simulink model "SPGF_FSK_0000_R2019b"  (R2019b)
settings: Solver=ode3  SolverName=ode4  StartTime=0.0  StopTime=1.4  FixedStep=50e-6/50  RelTol=1e-3  EnableMultiTasking=on
undefined symbols (not defined in the file): D11, Delta
libraries: powerlib x2544, powerlib_meascontrol x204, simulink x24
(part 14 of 33)

== system SPGF_FSK_0000_R2019b/W13/DPL ==
  Ccs2/1 : powerlib/Elements/Series RLC Branch  LConnTagsString=__new0  RConnTagsString=__new0  BranchType=R  Resistance=-Rg_matrix(3,4)*2  Inductance=1e-3  SetiL0=off  InitialCurrent=0  Capacitance=Rg_matrix(3,4)*2  Setx0=off  InitialVoltage=0  Measurements=None
  Ccs2/3 : powerlib/Elements/Series RLC Branch  LConnTagsString=__new0  RConnTagsString=__new0  BranchType=R  Resistance=-Rg_matrix(3,4)*2  Inductance=1e-3  SetiL0=off  InitialCurrent=0  Capacitance=Rg_matrix(3,4)*2  Setx0=off  InitialVoltage=0  Measurements=None
  Ccs3/1 : powerlib/Elements/Series RLC Branch  LConnTagsString=__new0  RConnTagsString=__new0  BranchType=R  Resistance=-Rg_matrix(5,6)*2  Inductance=1e-3  SetiL0=off  InitialCurrent=0  Capacitance=-C_matrix(5,6)/2  Setx0=off  InitialVoltage=0  Measurements=None
  Ccs3/3 : powerlib/Elements/Series RLC Branch  LConnTagsString=__new0  RConnTagsString=__new0  BranchType=R  Resistance=-Rg_matrix(5,6)*2  Inductance=1e-3  SetiL0=off  InitialCurrent=0  Capacitance=-C_matrix(5,6)/2  Setx0=off  InitialVoltage=0  Measurements=None
  DPL : powerlib/Elements/Distributed Parameters Line  Phases=6  Length=LineLength  Frequency=Frequency  Resistance=R_matrix  Inductance=L_matrix  Capacitance=C_matrix  x1=[-8.15e-05 -1.48873142828454 0 -11.7861642745277 0 4676.68792805612 0;-8.1e-05 -1.48913663578964 0 -11.7892921080622 0 4676.29069613494 0;-8.05e-05 -1.48954180655177 0 -11.7924196507075 0 4675.89334883091 0;-8e-05 -1.48994694056093 0 -11.7955469023866 0 4675.49588615384 0;-7.95e-05 -1.49035203780712 0 -11.7986738630222 0 4675.09830811353 0;-7.9e-05 -1.49075709828036 0 -11.8018005325372 0 4674.70061471979 0;-7.85e-05 -1.49116212197063 0 -11.8049269108544 0 4674.30280598244 0;-7.8e-05 -1.49156710886795 0 -11.8080529978968 0 4673.90488191129 0;-7.75e-05 -1.49197205896233 0 -11.8111787935871 0 4673.50684251616 0;-7.7e-05 -1.49237697224378 0 -11.8143042978483 0 4673.10868780687 0;-7.65e-05 -1.49278184870229 0 -11.8174295106032 0 4672.71041779325 0;-7.6e-05 -1.4931866883279 0 -11.8205544317747 0 4672.31203248511 0;-7.55e-05 -1.4935914911106 0 -11.8236790612857 0 4671.9135318923 0;-7.5e-05 -1.4939962570404 0 -11.8268033990591 0 4671.51491602465 0;-7.45e-05 -1.49440098610733 0 -11.8299274450179 0 4671.11618489198 0;-7.4e-05 -1.49480567830139 0 -11.8330511990848 0 4670.71733850414 0;-7.35e-05 -1.49521033361259 0 -11.836174661183 0 4670.31837687097 0;-7.3e-05 -1.49561495203097 0 -11.8392978312353 0 4669.91930000232 0;-7.25e-05 -1.49601953354652 0 -11.8424207091646 0 4669.52010790802 0;-7.2e-05 -1.49642407814927 0 -11.8455432948938 0 4669.12080059794 0;-7.15e-05 -1.49682858582923 0 -11.848665588346 0 4668.72137808191 0;-7.1e-05 -1.49723305657643 0 -11.8517875894441 0 4668.3218403698 0;-7.05e-05 -1.49763749038089 0 -11.8549092981111 0 4667.92218747147 0;-7e-05 -1.49804188723262 0 -11.8580307142699 0 4667.52241939678 0;-6.95e-05 -1.49844624712165 0 -11.8611518378435 0 4667.12253615559 0;-6.9e-05 -1.498850570038 0 -11.864272668755 0 4666.72253775776 0;-6.85e-05 -1.4992548559717 0 -11.8673932069272 0 4666.32242421317 0;-6.8e-05 -1.49965910491276 0 -11.8705134522833 0 4665.9221955317 0;-6.75e-05 -1.50006331685122 0 -11.8736334047461 0 4665.5218517232 0;-6.7e-05 -1.5004674917771 0 -11.8767530642388 0 4665.12139279757 0;-6.65e-05 -1.50087162968043 0 -11.8798724306844 0 4664.72081876468 0;-6.6e-05 -1.50127573055124 0 -11.8829915040059 0 4664.32012963442 0;-6.55e-05 -1.50167979437955 0 -11.8861102841263 0 4663.91932541667 0;-6.5e-05 -1.5020838211554 0 -11.8892287709687 0 4663.51840612133 0;-6.45e-05 -1.50248781086881 0 -11.8923469644561 0 4663.11737175828 0;-6.4e-05 -1.50289176350983 0 -11.8954648645117 0 4662.71622233743 0;-6.35e-05 -1.50329567906848 0 -11.8985824710584 0 4662.31495786866 0;-6.3e-05 -1.50369955753479 0 -11.9016997840193 0 4661.91357836188 0;-6.25e-05 -1.5041033988988 0 -11.9048168033176 0 4661.512083827 0;-6.2e-05 -1.50450720315056 0 -11.9079335288763 0 4661.11047427391 0;-6.15e-05 -1.50491097028008 0 -11.9110499606185 0 4660.70874971254 0;-6.1e-05 -1.50531470027741 0 -11.9141660984673 0 4660.30691015278 0;-6.05e-05 -1.50571839313259 0 -11.9172819423459 0 4659.90495560456 0;-6e-05 -1.50612204883566 0 -11.9203974921773 0 4659.5028860778 0;-5.95e-05 -1.50652566737666 0 -11.9235127478848 0 4659.10070158241 0;-5.9e-05 -1.50692924874563 0 -11.9266277093913 0 4658.69840212832 0;-5.85e-05 -1.50733279293261 0 -11.9297423766201 0 4658.29598772545 0;-5.8e-05 -1.50773629992764 0 -11.9328567494943 0 4657.89345838374 0;-5.75e-05 -1.50813976972077 0 -11.935970827937 0 4657.49081411311 0;-5.7e-05 -1.50854320230205 0 -11.9390846118715 0 4657.08805492351 0;-5.65e-05 -1.50894659766151 0 -11.9421981012209 0 4656.68518082486 0;-5.6e-05 -1.5093499557892 0 -11.9453112959083 0 4656.28219182711 0;-5.55e-05 -1.50975327667518 0 -11.948424195857 0 4655.8790879402 0;-5.5e-05 -1.51015656030949 0 -11.9515368009902 0 4655.47586917409 0;-5.45e-05 -1.51055980668219 0 -11.954649111231 0 4655.0725355387 0;-5.4e-05 -1.51096301578331 0 -11.9577611265026 0 4654.66908704401 0;-5.35e-05 -1.51136618760291 0 -11.9608728467284 0 4654.26552369996 0;-5.3e-05 -1.51176932213105 0 -11.9639842718314 0 4653.86184551652 0;-5.25e-05 -1.51217241935778 0 -11.9670954017349 0 ...(+8261 chars)]  x2=[-8.15e-05 -1.48162132976478 0 -11.6914851169798 0 4744.49609233801 0;-8.1e-05 -1.48204386266957 0 -11.694778370435 0 4744.09779479294 0;-8.05e-05 -1.48246635900639 0 -11.6980713353332 0 4743.69938019196 0;-8e-05 -1.48288881876481 0 -11.701364011593 0 4743.30084854488 0;-7.95e-05 -1.48331124193443 0 -11.7046563991333 0 4742.90219986155 0;-7.9e-05 -1.4837336285048 0 -11.7079484978727 0 4742.5034341518 0;-7.85e-05 -1.48415597846552 0 -11.7112403077301 0 4742.10455142546 0;-7.8e-05 -1.48457829180615 0 -11.7145318286242 0 4741.70555169239 0;-7.75e-05 -1.48500056851628 0 -11.7178230604738 0 4741.30643496242 0;-7.7e-05 -1.48542280858549 0 -11.7211140031977 0 4740.9072012454 0;-7.65e-05 -1.48584501200337 0 -11.7244046567148 0 4740.50785055119 0;-7.6e-05 -1.48626717875949 0 -11.7276950209437 0 4740.10838288964 0;-7.55e-05 -1.48668930884343 0 -11.7309850958034 0 4739.70879827059 0;-7.5e-05 -1.48711140224479 0 -11.7342748812126 0 4739.30909670393 0;-7.45e-05 -1.48753345895314 0 -11.7375643770902 0 4738.90927819949 0;-7.4e-05 -1.48795547895808 0 -11.7408535833549 0 4738.50934276716 0;-7.35e-05 -1.48837746224919 0 -11.7441424999258 0 4738.1092904168 0;-7.3e-05 -1.48879940881605 0 -11.7474311267215 0 4737.70912115827 0;-7.25e-05 -1.48922131864826 0 -11.750719463661 0 4737.30883500146 0;-7.2e-05 -1.48964319173541 0 -11.7540075106631 0 4736.90843195624 0;-7.15e-05 -1.49006502806709 0 -11.7572952676467 0 4736.50791203249 0;-7.1e-05 -1.49048682763288 0 -11.7605827345307 0 4736.10727524009 0;-7.05e-05 -1.49090859042239 0 -11.763869911234 0 4735.70652158893 0;-7e-05 -1.49133031642521 0 -11.7671567976753 0 4735.30565108889 0;-6.95e-05 -1.49175200563092 0 -11.7704433937737 0 4734.90466374987 0;-6.9e-05 -1.49217365802912 0 -11.7737296994481 0 4734.50355958176 0;-6.85e-05 -1.49259527360942 0 -11.7770157146173 0 4734.10233859446 0;-6.8e-05 -1.49301685236141 0 -11.7803014392004 0 4733.70100079787 0;-6.75e-05 -1.49343839427468 0 -11.7835868731161 0 4733.29954620188 0;-6.7e-05 -1.49385989933883 0 -11.7868720162835 0 4732.89797481641 0;-6.65e-05 -1.49428136754348 0 -11.7901568686214 0 4732.49628665136 0;-6.6e-05 -1.4947027988782 0 -11.7934414300489 0 4732.09448171665 0;-6.55e-05 -1.49512419333261 0 -11.7967257004849 0 4731.69256002219 0;-6.5e-05 -1.49554555089632 0 -11.8000096798484 0 4731.29052157789 0;-6.45e-05 -1.49596687155891 0 -11.8032933680583 0 4730.88836639368 0;-6.4e-05 -1.49638815531 0 -11.8065767650336 0 4730.48609447948 0;-6.35e-05 -1.49680940213919 0 -11.8098598706933 0 4730.08370584521 0;-6.3e-05 -1.4972306120361 0 -11.8131426849564 0 4729.6812005008 0;-6.25e-05 -1.49765178499031 0 -11.8164252077419 0 4729.27857845619 0;-6.2e-05 -1.49807292099146 0 -11.8197074389688 0 4728.87583972131 0;-6.15e-05 -1.49849402002913 0 -11.8229893785561 0 4728.47298430609 0;-6.1e-05 -1.49891508209295 0 -11.8262710264228 0 4728.07001222048 0;-6.05e-05 -1.49933610717251 0 -11.829552382488 0 4727.66692347442 0;-6e-05 -1.49975709525745 0 -11.8328334466706 0 4727.26371807785 0;-5.95e-05 -1.50017804633736 0 -11.8361142188898 0 4726.86039604073 0;-5.9e-05 -1.50059896040186 0 -11.8393946990646 0 4726.456957373 0;-5.85e-05 -1.50101983744056 0 -11.8426748871141 0 4726.05340208462 0;-5.8e-05 -1.50144067744309 0 -11.8459547829572 0 4725.64973018554 0;-5.75e-05 -1.50186148039905 0 -11.8492343865132 0 4725.24594168573 0;-5.7e-05 -1.50228224629806 0 -11.852513697701 0 4724.84203659516 0;-5.65e-05 -1.50270297512975 0 -11.8557927164397 0 4724.43801492378 0;-5.6e-05 -1.50312366688373 0 -11.8590714426485 0 4724.03387668156 0;-5.55e-05 -1.50354432154961 0 -11.8623498762464 0 4723.62962187848 0;-5.5e-05 -1.50396493911703 0 -11.8656280171526 0 4723.22525052451 0;-5.45e-05 -1.5043855195756 0 -11.8689058652861 0 4722.82076262963 0;-5.4e-05 -1.50480606291495 0 -11.8721834205661 0 4722.41615820382 0;-5.35e-05 -1.50522656912469 0 -11.8754606829118 0 4722.01143725705 0;-5.3e-05 -1.50564703819446 0 -11.8787376522422 0 4721.60659979933 0;-5.25e-05 -1.50606747011388 0 -11.8820143284765 0 ...(+8265 chars)]  x3=[-8.15e-05 0.0158008018941895 0 -0.497557667568893 0 442.095796396926 0;-8.1e-05 0.0157969192286376 0 -0.497893185344398 0 442.062522662758 0;-8.05e-05 0.0157930361733123 0 -0.498228690834881 0 442.029238021135 0;-8e-05 0.0157891527283095 0 -0.498564184032065 0 441.995942472877 0;-7.95e-05 0.015785268893725 0 -0.49889966492767 0 441.962636018807 0;-7.9e-05 0.0157813846696546 0 -0.499235133513419 0 441.929318659746 0;-7.85e-05 0.0157775000561941 0 -0.499570589781035 0 441.895990396516 0;-7.8e-05 0.0157736150534395 0 -0.499906033722241 0 441.86265122994 0;-7.75e-05 0.0157697296614864 0 -0.50024146532876 0 441.82930116084 0;-7.7e-05 0.0157658438804309 0 -0.500576884592316 0 441.795940190038 0;-7.65e-05 0.0157619577103688 0 -0.500912291504632 0 441.762568318359 0;-7.6e-05 0.015758071151396 0 -0.501247686057433 0 441.729185546626 0;-7.55e-05 0.0157541842036083 0 -0.501583068242443 0 441.695791875661 0;-7.5e-05 0.0157502968671017 0 -0.501918438051386 0 441.66238730629 0;-7.45e-05 0.0157464091419722 0 -0.502253795475989 0 441.628971839336 0;-7.4e-05 0.0157425210283155 0 -0.502589140507976 0 441.595545475624 0;-7.35e-05 0.0157386325262278 0 -0.502924473139073 0 441.562108215979 0;-7.3e-05 0.0157347436358048 0 -0.503259793361006 0 441.528660061225 0;-7.25e-05 0.0157308543571426 0 -0.503595101165502 0 441.495201012189 0;-7.2e-05 0.0157269646903371 0 -0.503930396544286 0 441.461731069695 0;-7.15e-05 0.0157230746354844 0 -0.504265679489086 0 441.42825023457 0;-7.1e-05 0.0157191841926803 0 -0.50460094999163 0 441.394758507639 0;-7.05e-05 0.0157152933620208 0 -0.504936208043644 0 441.361255889729 0;-7e-05 0.0157114021436021 0 -0.505271453636856 0 441.327742381666 0;-6.95e-05 0.0157075105375201 0 -0.505606686762995 0 441.294217984278 0;-6.9e-05 0.0157036185438707 0 -0.505941907413789 0 441.260682698391 0;-6.85e-05 0.0156997261627502 0 -0.506277115580967 0 441.227136524834 0;-6.8e-05 0.0156958333942544 0 -0.506612311256258 0 441.193579464433 0;-6.75e-05 0.0156919402384794 0 -0.506947494431392 0 441.160011518018 0;-6.7e-05 0.0156880466955213 0 -0.507282665098097 0 441.126432686415 0;-6.65e-05 0.0156841527654762 0 -0.507617823248104 0 441.092842970454 0;-6.6e-05 0.0156802584484402 0 -0.507952968873143 0 441.059242370963 0;-6.55e-05 0.0156763637445092 0 -0.508288101964946 0 441.025630888772 0;-6.5e-05 0.0156724686537795 0 -0.508623222515242 0 440.992008524709 0;-6.45e-05 0.0156685731763472 0 -0.508958330515763 0 440.958375279605 0;-6.4e-05 0.0156646773123082 0 -0.509293425958241 0 440.924731154289 0;-6.35e-05 0.0156607810617589 0 -0.509628508834407 0 440.891076149591 0;-6.3e-05 0.0156568844247953 0 -0.509963579135993 0 440.857410266342 0;-6.25e-05 0.0156529874015135 0 -0.510298636854733 0 440.823733505372 0;-6.2e-05 0.0156490899920098 0 -0.510633681982359 0 440.790045867513 0;-6.15e-05 0.0156451921963803 0 -0.510968714510603 0 440.756347353596 0;-6.1e-05 0.0156412940147211 0 -0.5113037344312 0 440.722637964451 0;-6.05e-05 0.0156373954471284 0 -0.511638741735883 0 440.688917700911 0;-6e-05 0.0156334964936985 0 -0.511973736416386 0 440.655186563808 0;-5.95e-05 0.0156295971545275 0 -0.512308718464444 0 440.621444553975 0;-5.9e-05 0.0156256974297116 0 -0.51264368787179 0 440.587691672242 0;-5.85e-05 0.0156217973193472 0 -0.512978644630161 0 440.553927919445 0;-5.8e-05 0.0156178968235303 0 -0.513313588731291 0 440.520153296415 0;-5.75e-05 0.0156139959423573 0 -0.513648520166916 0 440.486367803985 0;-5.7e-05 0.0156100946759244 0 -0.513983438928771 0 440.452571442991 0;-5.65e-05 0.0156061930243278 0 -0.514318345008594 0 440.418764214265 0;-5.6e-05 0.0156022909876638 0 -0.51465323839812 0 440.384946118641 0;-5.55e-05 0.0155983885660288 0 -0.514988119089086 0 440.351117156954 0;-5.5e-05 0.0155944857595189 0 -0.51532298707323 0 440.317277330039 0;-5.45e-05 0.0155905825682305 0 -0.515657842342289 0 440.283426638731 0;-5.4e-05 0.01558667899226 0 -0.515992684888001 0 440.249565083865 0;-5.35e-05 0.0155827750317035 0 -0.516327514702103 0 440.215692666276 0 ...(+8595 chars)]  x4=[-8.15e-05 -0.0346768728477826 0 -0.849228754042194 0 337.992547305937 0;-8.1e-05 -0.0346784108319786 0 -0.849263980666828 0 337.960266140897 0;-8.05e-05 -0.0346799479605192 0 -0.849299186336713 0 337.927976637021 0;-8e-05 -0.0346814842333663 0 -0.84933437105098 0 337.895678795107 0;-7.95e-05 -0.0346830196504821 0 -0.849369534808762 0 337.863372615951 0;-7.9e-05 -0.0346845542118287 0 -0.849404677609191 0 337.831058100351 0;-7.85e-05 -0.0346860879173683 0 -0.849439799451399 0 337.798735249104 0;-7.8e-05 -0.0346876207670629 0 -0.849474900334521 0 337.766404063006 0;-7.75e-05 -0.0346891527608748 0 -0.849509980257689 0 337.734064542857 0;-7.7e-05 -0.0346906838987662 0 -0.849545039220039 0 337.701716689454 0;-7.65e-05 -0.0346922141806992 0 -0.849580077220706 0 337.669360503595 0;-7.6e-05 -0.0346937436066362 0 -0.849615094258824 0 337.636995986078 0;-7.55e-05 -0.0346952721765394 0 -0.84965009033353 0 337.604623137703 0;-7.5e-05 -0.034696799890371 0 -0.84968506544396 0 337.572241959267 0;-7.45e-05 -0.0346983267480934 0 -0.849720019589252 0 337.53985245157 0;-7.4e-05 -0.0346998527496689 0 -0.849754952768543 0 337.507454615411 0;-7.35e-05 -0.0347013778950599 0 -0.849789864980971 0 337.47504845159 0;-7.3e-05 -0.0347029021842287 0 -0.849824756225674 0 337.442633960905 0;-7.25e-05 -0.0347044256171377 0 -0.849859626501792 0 337.410211144157 0;-7.2e-05 -0.0347059481937494 0 -0.849894475808464 0 337.377780002146 0;-7.15e-05 -0.0347074699140261 0 -0.849929304144831 0 337.345340535672 0;-7.1e-05 -0.0347089907779302 0 -0.849964111510033 0 337.312892745535 0;-7.05e-05 -0.0347105107854244 0 -0.849998897903211 0 337.280436632537 0;-7e-05 -0.0347120299364711 0 -0.850033663323506 0 337.247972197477 0;-6.95e-05 -0.0347135482310327 0 -0.850068407770062 0 337.215499441157 0;-6.9e-05 -0.0347150656690719 0 -0.850103131242021 0 337.183018364378 0;-6.85e-05 -0.0347165822505512 0 -0.850137833738526 0 337.150528967941 0;-6.8e-05 -0.0347180979754331 0 -0.85017251525872 0 337.118031252649 0;-6.75e-05 -0.0347196128436803 0 -0.850207175801749 0 337.085525219303 0;-6.7e-05 -0.0347211268552554 0 -0.850241815366756 0 337.053010868704 0;-6.65e-05 -0.034722640010121 0 -0.850276433952888 0 337.020488201656 0;-6.6e-05 -0.0347241523082399 0 -0.850311031559289 0 336.987957218961 0;-6.55e-05 -0.0347256637495746 0 -0.850345608185107 0 336.955417921421 0;-6.5e-05 -0.0347271743340879 0 -0.850380163829488 0 336.92287030984 0;-6.45e-05 -0.0347286840617425 0 -0.850414698491579 0 336.89031438502 0;-6.4e-05 -0.0347301929325012 0 -0.850449212170529 0 336.857750147765 0;-6.35e-05 -0.0347317009463268 0 -0.850483704865486 0 336.825177598878 0;-6.3e-05 -0.0347332081031819 0 -0.850518176575598 0 336.792596739162 0;-6.25e-05 -0.0347347144030296 0 -0.850552627300016 0 336.760007569423 0;-6.2e-05 -0.0347362198458324 0 -0.850587057037888 0 336.727410090463 0;-6.15e-05 -0.0347377244315535 0 -0.850621465788367 0 336.694804303088 0;-6.1e-05 -0.0347392281601555 0 -0.850655853550602 0 336.662190208101 0;-6.05e-05 -0.0347407310316014 0 -0.850690220323745 0 336.629567806308 0;-6e-05 -0.0347422330458542 0 -0.850724566106948 0 336.596937098513 0;-5.95e-05 -0.0347437342028767 0 -0.850758890899365 0 336.564298085522 0;-5.9e-05 -0.0347452345026319 0 -0.850793194700146 0 336.531650768139 0;-5.85e-05 -0.0347467339450829 0 -0.850827477508448 0 336.498995147171 0;-5.8e-05 -0.0347482325301925 0 -0.850861739323423 0 336.466331223423 0;-5.75e-05 -0.0347497302579239 0 -0.850895980144226 0 336.433658997701 0;-5.7e-05 -0.03475122712824 0 -0.850930199970012 0 336.400978470811 0;-5.65e-05 -0.034752723141104 0 -0.850964398799937 0 336.36828964356 0;-5.6e-05 -0.034754218296479 0 -0.850998576633157 0 336.335592516754 0;-5.55e-05 -0.0347557125943279 0 -0.851032733468829 0 336.3028870912 0;-5.5e-05 -0.034757206034614 0 -0.85106686930611 0 336.270173367704 0;-5.45e-05 -0.0347586986173005 0 -0.851100984144158 0 336.237451347075 0;-5.4e-05 -0.0347601903423504 0 -0.851135077982131 0 336.204721030119 0;-5.35e-05 ...(+8736 chars)]  x5=8.10078942075617e-05  V1=ones(3,3)  V2=ones(3,3)  I1=ones(3,3)  I2=ones(3,3)  nHarmo=1  Measurements=None  Decoupling=off  VsMag0=0  VrMag0=0  VsAngle0=0  VrAngle0=0  IsMag0=0  IrMag0=0  IsAngle0=0  IrAngle0=0
  Ground{1..4} (4 alike) : powerlib/Elements/Ground  LConnTagsString=a
  Rcs*1 : powerlib/Elements/Series RLC Branch  LConnTagsString=__new0  RConnTagsString=__new0  BranchType=R  Resistance=-Rg_matrix(1,2)*2  Inductance=1e-3  SetiL0=off  InitialCurrent=0  Capacitance=Rg_matrix(1,2)*2  Setx0=off  InitialVoltage=0  Measurements=None
  Rcs*2 : powerlib/Elements/Series RLC Branch  LConnTagsString=__new0  RConnTagsString=__new0  BranchType=R  Resistance=-Rg_matrix(1,2)*2  Inductance=1e-3  SetiL0=off  InitialCurrent=0  Capacitance=Rg_matrix(1,2)*2  Setx0=off  InitialVoltage=0  Measurements=None
  Rgsg1/1 : powerlib/Elements/Series RLC Branch  LConnTagsString=__new0  RConnTagsString=__new0  BranchType=R  Resistance=(Rg_matrix(4,4)+Rg_matrix(3,4))*2  Inductance=1e-3  SetiL0=off  InitialCurrent=0  Capacitance=Rg_matrix(1,2)*2  Setx0=off  InitialVoltage=0  Measurements=None
  Rgsg1/2 : powerlib/Elements/Series RLC Branch  LConnTagsString=__new0  RConnTagsString=__new0  BranchType=R  Resistance=(Rg_matrix(2,2)+Rg_matrix(1,2))*2  Inductance=1e-3  SetiL0=off  InitialCurrent=0  Capacitance=Rg_matrix(1,2)*2  Setx0=off  InitialVoltage=0  Measurements=None
  Rgsg1/3 : powerlib/Elements/Series RLC Branch  LConnTagsString=__new0  RConnTagsString=__new0  BranchType=R  Resistance=(Rg_matrix(4,4)+Rg_matrix(3,4))*2  Inductance=1e-3  SetiL0=off  InitialCurrent=0  Capacitance=Rg_matrix(1,2)*2  Setx0=off  InitialVoltage=0  Measurements=None
  Rgsg1/4 : powerlib/Elements/Series RLC Branch  LConnTagsString=__new0  RConnTagsString=__new0  BranchType=R  Resistance=(Rg_matrix(2,2)+Rg_matrix(1,2))*2  Inductance=1e-3  SetiL0=off  InitialCurrent=0  Capacitance=Rg_matrix(1,2)*2  Setx0=off  InitialVoltage=0  Measurements=None
  Rsg*1 : powerlib/Elements/Series RLC Branch  LConnTagsString=__new0  RConnTagsString=__new0  BranchType=R  Resistance=(Rg_matrix(6,6)+Rg_matrix(5,6))*2  Inductance=1e-3  SetiL0=off  InitialCurrent=0  Capacitance=Rg_matrix(1,2)*2  Setx0=off  InitialVoltage=0  Measurements=None
  Rsg*2 : powerlib/Elements/Series RLC Branch  LConnTagsString=__new0  RConnTagsString=__new0  BranchType=R  Resistance=(Rg_matrix(6,6)+Rg_matrix(5,6))*2  Inductance=1e-3  SetiL0=off  InitialCurrent=0  Capacitance=Rg_matrix(1,2)*2  Setx0=off  InitialVoltage=0  Measurements=None
  A : PMIOPort  Side=Left
  B : PMIOPort  Port=2  Side=Left
  C : PMIOPort  Port=3  Side=Left
  a : PMIOPort  Port=4  Side=Right
  b : PMIOPort  Port=5  Side=Right
  c : PMIOPort  Port=6  Side=Right
  connections:
  c/RConn1 -- Ccs3/1/RConn1 -- DPL/RConn5
  b/RConn1 -- Ccs2/1/RConn1 -- DPL/RConn3
  a/RConn1 -- DPL/RConn1 -- Rcs*1/RConn1
  Ground4/LConn1 -- DPL/RConn6 -- Ccs3/1/LConn1 -- Rsg*1/LConn1 -- Rcs*1/LConn1 -- Rgsg1/4/LConn1 -- DPL/RConn2 -- DPL/RConn4 -- Ccs2/1/LConn1 -- Rgsg1/3/LConn1
  Ground1/LConn1 -- Rgsg1/4/RConn1 -- Rsg*1/RConn1 -- Rgsg1/3/RConn1
  Ground3/LConn1 -- Ccs3/3/LConn1 -- Rsg*2/LConn1 -- DPL/LConn6 -- Rgsg1/1/LConn1 -- Ccs2/3/LConn1 -- DPL/LConn4 -- Rgsg1/2/LConn1 -- Rcs*2/LConn1 -- DPL/LConn2
  Ground2/LConn1 -- Rgsg1/1/RConn1 -- Rsg*2/RConn1 -- Rgsg1/2/RConn1
  Ccs3/3/RConn1 -- DPL/LConn5 -- C/RConn1
  Ccs2/3/RConn1 -- DPL/LConn3 -- B/RConn1
  Rcs*2/RConn1 -- DPL/LConn1 -- A/RConn1
